simulink model "batt_shutdown"  (R2013a)
settings: Solver=ode45  StartTime=0.0  StopTime=10.0  RelTol=1e-3
libraries: fl_lib x8, simulink x1, nesl_utility x1
settings Model: Creator=Suddenlink  LastModifiedBy=Suddenlink

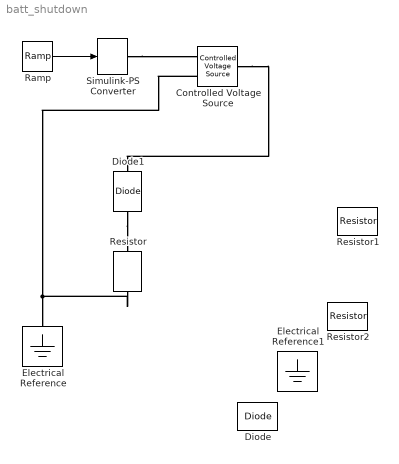
== system batt_shutdown ==
  Controlled Voltage Source : fl_lib/Electrical/Electrical Sources/Controlled Voltage Source  i_Log=off  v_Log=off  LocalVarNames=|i|v  LocalVarDescs=|i|v  LocalVarLogging=[0 0]
  Diode : fl_lib/Electrical/Electrical Elements/Diode  Vf=0.6 V  Ron=0.3 Ohm  Goff=1e-8 1/Ohm  i_Log=off  v_Log=off  LocalVarNames=|i|v  LocalVarDescs=|i|v  LocalVarLogging=[0 0]
  Diode1 : fl_lib/Electrical/Electrical Elements/Diode  Vf=0.6 V  Ron=0.3 Ohm  Goff=1e-8 1/Ohm  i_Log=off  v_Log=off  LocalVarNames=|i|v  LocalVarDescs=|i|v  LocalVarLogging=[0 0]
  Electrical Reference : fl_lib/Electrical/Electrical Elements/Electrical Reference  i_Log=off  LocalVarNames=|i  LocalVarDescs=|i  LocalVarLogging=0
  Electrical Reference1 : fl_lib/Electrical/Electrical Elements/Electrical Reference  i_Log=off  LocalVarNames=|i  LocalVarDescs=|i  LocalVarLogging=0
  Ramp : simulink/Sources/Ramp  slope=1  start=0  X0=0
  Resistor : fl_lib/Electrical/Electrical Elements/Resistor  R=1 Ohm  i_Log=off  v_Log=off  LocalVarNames=|i|v  LocalVarDescs=|i|v  LocalVarLogging=[0 0]
  Resistor1 : fl_lib/Electrical/Electrical Elements/Resistor  R=1 Ohm  i_Log=off  v_Log=off  LocalVarNames=|i|v  LocalVarDescs=|i|v  LocalVarLogging=[0 0]
  Resistor2 : fl_lib/Electrical/Electrical Elements/Resistor  R=1 Ohm  i_Log=off  v_Log=off  LocalVarNames=|i|v  LocalVarDescs=|i|v  LocalVarLogging=[0 0]
  Simulink-PS Converter : nesl_utility/Simulink-PS Converter  PhysicalDomain=network_engine_domain  SubClassName=ps_input  LeftPortType=input  RightPortType=output  PseudoPeriodic=off  Frequencies=[]  NoiseDistribution=none  NoiseParameters=[]  Unit=1  AffineConversion=off  InputFiltering=off  SimscapeFilterOrder=1  InputFilterTimeConstant=0.001  UdotUserProvided=1
  wires:
  Ramp/1 -> Simulink-PS Converter/1
  connections:
  Simulink-PS Converter/RConn1 -- Controlled Voltage Source/RConn1
  Controlled Voltage Source/RConn2 -- Resistor/RConn1 -- Electrical Reference/LConn1
  Diode1/RConn1 -- Resistor/LConn1
  Controlled Voltage Source/LConn1 -- Diode1/LConn1
